simulink model "Spike_Generator_matt"  (R2019b)
settings: Solver=VariableStepAuto  StartTime=0.0  StopTime=testtime  RelTol=1e-3
InitFcn:
  | Spike_Generator_Test_Parameters
StopFcn:
  | Verify_Spike_Generator
values from neighbouring files (symbols this model uses):
  Fs = 48e3    (= 48000)    [Spike_Generator_Test_Parameters.m]    (also in modelparameters.m)
  nSites = 4    [Spike_Generator_Test_Parameters.m]
  tabs = 0.6e-3    (= 0.0006)    [Spike_Generator_Test_Parameters.m]
  trel = 0.6e-3    (= 0.0006)    [Spike_Generator_Test_Parameters.m]
libraries: dspsrcs4 x4
(part 2 of 3)

== stateflow chart Spike_Generator_matt/Spike Generator Singles/Stateflow Logic Chart ==
  settings: updateMethod=DISCRETE  sampleTime=tdres  executeAtInitialization=1
  note: 1st Synaptic Site State
      |
      | - Updates according to whether the synaptic site is sensing input or is going through the redocking period.
  note: 2nd Synaptic Site State
      |
      | - Updates according to whether the synaptic site is sensing input or is going through the redocking period.
  note: 3rd Synaptic Site State
      |
      | - Updates according to whether the synaptic site is sensing input or is going through the redocking period.
  note: 4th Synaptic Site State
      |
      | - Updates according to whether the synaptic site is sensing input or is going through the redocking period.
  note: Redocking Decay State
      |
      | - Updates according to whether the redocking period should be decayed or a redocking event has occured during the time step
  note: Synaptic State
      |
      | - Updates according to whether the synapse is ready to fire or is going through the refractory period.
  state SynapticSite1 [parallel]
    settings: executionOrder=2
    note: Synaptic Site Sensing Input
    note: Synaptic Site In Redocking Period
    note: Default Transition
    state SenseInput
      entry:
      SredockStatus1 = single(0);
      SXsum1 = SXsum1 + synout/(single(4));
      SreleaseStatus1 = checkRelease(SXsum1, SunitRateInterval1);
      during:
      SXsum1 = SXsum1 + synout/(single(4));
      SreleaseStatus1 = checkRelease(SXsum1, SunitRateInterval1);
      exit:
      SoneSiteRedock1 = getNewRedock(Scurrent_redocking_period, randNums);
      SXsum1= single(0);
      SunitRateInterval1 = getNewUnitRateInterval(randNums);
    state RedockPeriod
      entry:
      Selapsed_time1 = single(0);
      SredockStatus1 = checkRedock(Selapsed_time1, SoneSiteRedock1);
      Selapsed_time1  = Selapsed_time1 + Stdres;
      SreleaseStatus1 = single(0);
      during:
      SredockStatus1 = checkRedock(Selapsed_time1, SoneSiteRedock1);
      Selapsed_time1 = Selapsed_time1 + Stdres;
      exit:
      Selapsed_time1 = single(0);
      Scurrent_redocking_period = Sprevious_redocking_period + St_rd_jump;
      Sprevious_redocking_period = Scurrent_redocking_period;
    (default) -> SynapticSite1.RedockPeriod
    SynapticSite1.SenseInput -> SynapticSite1.RedockPeriod : [SreleaseStatus1 == single(1)]
    SynapticSite1.RedockPeriod -> SynapticSite1.SenseInput : [SredockStatus1 == single(1)]
  state SynapticSite2 [parallel]
    settings: executionOrder=3
    note: Synaptic Site Sensing Input
    note: Synaptic Site In Redocking Period
    note: Default Transition
    state SenseInput
      entry:
      SredockStatus2 = single(0);
      SXsum2 = SXsum2 + synout/(single(4));
      SreleaseStatus2 = checkRelease(SXsum2, SunitRateInterval2);
      during:
      SXsum2 = SXsum2 + synout/(single(4));
      SreleaseStatus2 = checkRelease(SXsum2, SunitRateInterval2);
      exit:
      SoneSiteRedock2 = getNewRedock(Scurrent_redocking_period, randNums);
      SXsum2= single(0);
      SunitRateInterval2 = getNewUnitRateInterval(randNums);
    state RedockPeriod
      entry:
      Selapsed_time2 = single(0);
      SredockStatus2 = checkRedock(Selapsed_time2, SoneSiteRedock2);
      Selapsed_time2  = Selapsed_time2 + Stdres;
      SreleaseStatus2 = single(0);
      during:
      SredockStatus2 = checkRedock(Selapsed_time2, SoneSiteRedock2);
      Selapsed_time2 = Selapsed_time2 + Stdres;
      exit:
      Selapsed_time2 = single(0);
      Scurrent_redocking_period = Sprevious_redocking_period + St_rd_jump;
      Sprevious_redocking_period = Scurrent_redocking_period;
    (default) -> SynapticSite2.RedockPeriod
    SynapticSite2.SenseInput -> SynapticSite2.RedockPeriod : [SreleaseStatus2 == single(1)]
    SynapticSite2.RedockPeriod -> SynapticSite2.SenseInput : [SredockStatus2 == single(1)]
  state SynapticSite3 [parallel]
    settings: executionOrder=4
    note: Synaptic Site Sensing Input
    note: Synaptic Site In Redocking Period
    note: Default Transition
    state SenseInput
      entry:
      SredockStatus3 = single(0);
      SXsum3 = SXsum3 + synout/(single(4));
      SreleaseStatus3 = checkRelease(SXsum3, SunitRateInterval3);
      during:
      SXsum3 = SXsum3 + synout/(single(4));
      SreleaseStatus3 = checkRelease(SXsum3, SunitRateInterval3);
      exit:
      SoneSiteRedock3 = getNewRedock(Scurrent_redocking_period, randNums);
      SXsum3= single(0);
      SunitRateInterval3 = getNewUnitRateInterval(randNums);
    state RedockPeriod
      entry:
      Selapsed_time3 = single(0);
      SredockStatus3 = checkRedock(Selapsed_time3, SoneSiteRedock3);
      Selapsed_time3  = Selapsed_time3 + Stdres;
      SreleaseStatus3 = single(0);
      during:
      SredockStatus3 = checkRedock(Selapsed_time3, SoneSiteRedock3);
      Selapsed_time3 = Selapsed_time3 + Stdres;
      exit:
      Selapsed_time3 = single(0);
      Scurrent_redocking_period = Sprevious_redocking_period + St_rd_jump;
      Sprevious_redocking_period = Scurrent_redocking_period;
    (default) -> SynapticSite3.RedockPeriod
    SynapticSite3.SenseInput -> SynapticSite3.RedockPeriod : [SreleaseStatus3 == single(1)]
    SynapticSite3.RedockPeriod -> SynapticSite3.SenseInput : [SredockStatus3 == single(1)]
  state SynapticSite4 [parallel]
    settings: executionOrder=5
    note: Synaptic Site Sensing Input
    note: Synaptic Site In Redocking Period
    note: Default Transition
    state SenseInput
      entry:
      SredockStatus4 = single(0);
      SXsum4 = SXsum4 + synout/(single(4));
      SreleaseStatus4 = checkRelease(SXsum4, SunitRateInterval4);
      during:
      SXsum4 = SXsum4 + synout/(single(4));
      SreleaseStatus4 = checkRelease(SXsum4, SunitRateInterval4);
      exit:
      SoneSiteRedock4 = getNewRedock(Scurrent_redocking_period, randNums);
      SXsum4= single(0);
      SunitRateInterval4 = getNewUnitRateInterval(randNums);
    state RedockPeriod
      entry:
      Selapsed_time4 = single(0);
      SredockStatus4 = checkRedock(Selapsed_time4, SoneSiteRedock4);
      Selapsed_time4  = Selapsed_time4 + Stdres;
      SreleaseStatus4 = single(0);
      during:
      SredockStatus4 = checkRedock(Selapsed_time4, SoneSiteRedock4);
      Selapsed_time4 = Selapsed_time4 + Stdres;
      exit:
      Selapsed_time4 = single(0);
      Scurrent_redocking_period = Sprevious_redocking_period + St_rd_jump;
      Sprevious_redocking_period = Scurrent_redocking_period;
    (default) -> SynapticSite4.RedockPeriod
    SynapticSite4.SenseInput -> SynapticSite4.RedockPeriod : [SreleaseStatus4 == single(1)]
    SynapticSite4.RedockPeriod -> SynapticSite4.SenseInput : [SredockStatus4 == single(1)]
  state RedockingDecay [parallel]
    settings: executionOrder=6
    note: Decay Redocking Period
    note: Don't Decay Redocking Period
    note: Default Transition
    state DecayRedockingPeriod
      entry:
      Scurrent_redocking_period = decayRedock(Sprevious_redocking_period, Stdres, Stau, St_rd_rest);
      Sprevious_redocking_period = Scurrent_redocking_period;
      Strd_vector = Scurrent_redocking_period;
      during:
      Scurrent_redocking_period = decayRedock(Sprevious_redocking_period, Stdres, Stau, St_rd_rest);
      Sprevious_redocking_period = Scurrent_redocking_period;
      Strd_vector = Scurrent_redocking_period;
    state NoDecay
      entry:
      Strd_vector = Scurrent_redocking_period;
      during:
      Strd_vector = Scurrent_redocking_period;
    (default) -> DecayRedockingPeriod
    DecayRedockingPeriod -> NoDecay : [SredockStatus1 == single(1) || SredockStatus2 == single(1) || SredockStatus3 == single(1) || SredockStatus4 == single(1)]
    NoDecay -> DecayRedockingPeriod : [SredockStatus1 == single(0) && SredockStatus2 == single(0) && SredockStatus3 == single(0) && SredockStatus4 == single(0)]
  state Synapse [parallel]
    settings: executionOrder=1
    note: Synapse Ready to Fire
    note: Synapse in Refractory Period
    note: Default Transition
    state RefractoryPeriod
      entry:
      SrefractoryStatus = checkRefractory(Srefractory_time, STref);
      Srefractory_time = Srefractory_time + Stdres;
      during:
      Ssptime = single(0);
      SrefractoryStatus = checkRefractory(Srefractory_time, STref);
      Srefractory_time = Srefractory_time + Stdres;
      exit:
      Srefractory_time = single(0);
      Ssptime = single(0);
    state SynapseReady
      during:
      Ssptime = single(0);
      exit:
      Ssptime = single(1);
      SspCount = SspCount + single(1);
      STref = getTref(synout, randNums, Strel, Stabs);
    (default) -> SynapseReady
    SynapseReady -> RefractoryPeriod : [SreleaseStatus1 == single(1) || SreleaseStatus2 == single(1) || SreleaseStatus3 == single(1) || SreleaseStatus4 == single(1)]
    RefractoryPeriod -> SynapseReady : [SrefractoryStatus == single(0)]
  note: Release Status Graphical Function
      |
      | Input : Sensing Input Sum (Xsum) & Release Threshold (unitRateInterval)
      |
      | Output : Release Status Condition (releaseStatus)
      |
      | - Checks if a Release Event Occurs for the Synaptic Site (1) or not (0)
  state releaseStatuscond = checkRelease(Xsumval, unitRateIntervalval) [function]
    (default) -> (junction 138) : % Check to see if a release event occurs.
    (junction 138) -> (junction 139) [order 1] : [Xsumval >= unitRateIntervalval]
    (junction 138) -> (junction 140) [order 2] : {releaseStatuscond = single(0);}
    (junction 139) -> (junction 141) : {releaseStatuscond = single(1);}
    (junction 141) -> (junction 140)
    (junction 140) -> (junction 142)
  state redockStatuscond = checkRedock(elapsed_timeval, oneSiteRedockval) [function]
    (default) -> (junction 153) : % Check to see if a redocking event occurs.
    (junction 153) -> (junction 154) [order 1] : [elapsed_timeval >= oneSiteRedockval]
    (junction 153) -> (junction 155) [order 2] : {redockStatuscond = single(0);}
    (junction 154) -> (junction 156) : {redockStatuscond = single(1);}
    (junction 156) -> (junction 155)
    (junction 155) -> (junction 157)
  note: Redock Status Graphical Function
      |
      | Input : Elapsed Time during Redocking Event (elapsed_time) & Site Specific Redocking Period (oneSiteRedock)
      |
      | Output : Redock Status Condition (redockStatus)
      |
      | - Checks if a Redocking Event Occurs for the Synaptic Site (1) or not (0)
  state refractoryStatuscond = checkRefractory(refractory_timeval, Trefval) [function]
    (default) -> (junction 272) : % Check to see if the synapse is in the refractory period.
    (junction 272) -> (junction 273) [order 1] : [refractory_timeval >= Trefval]
    (junction 272) -> (junction 274) [order 2] : {refractoryStatuscond = single(1);}
    (junction 273) -> (junction 275) : {refractoryStatuscond = single(0);}
    (junction 275) -> (junction 274)
    (junction 274) -> (junction 276)
  note: Refractory Status Graphical Function
      |
      | Input : Elapsed Time during Refractory Period (refractory_time) & Refractory Period (Tref)
      |
      | Output : Refractory Status Condition (refractoryStatus)
      |
      | - Checks if the Synapse is in the Refractory Period (1) or not (0)
  note: Get New Unit Rate Interval MATLAB Function
      |
      | Input : Uniformly Distributed Random Number between 0 and 1 (randNums)
      |
      | Output : New Release Threshold Value (unitRateInterval)
      |
      | - Calculates the New Release Threshold Value for the Synaptic Site after a Release Event
  note: Get New Site Specific Redocking Period MATLAB Function
      |
      | Input : Current Redocking Period (current_redocking_period) & Uniformly Distributed Random Number between 0 and 1 (randNums)
      |
      | Output : New Redocking Period for Specific Synaptic Site (oneSiteRedock)
      |
      | - Calculates the New Redocking Period for Specific Synaptic Site
  note: Decay Redocking Period MATLAB Function
      |
      | Input : Previous Redocking Period (previous_redocking_period), Sample Time (tdres),
      | Decay Time Constant (tau), & Resting Redocking Time (t_rd_rest)
      |
      | Output : Current Redocking Period (current_redocking_period)
      |
      | - Decays the Redocking Period for the Next TIme Step
  note: Get New Refractory Period MATLAB Function
      |
      | Input : Synapse Output (synout), Uniformly Distributed Random Number between 0 and 1 (randNums),
      | Relative Refractory Time (trel), & Absolute Refractory Time (tabs)
      |
      | Output : New Refractory Period for the Synapse (Tref)
      |
      | - Calculates the New Refractory Period for the Synapse
  data: Xsumval function_input single; releaseStatuscond function_output single; unitRateIntervalval function_input single; elapsed_timeval function_input single; redockStatuscond function_output single; oneSiteRedockval function_input single; refractory_timeval function_input single; refractoryStatuscond function_output single; Trefval function_input single; randNumsval function_input single; unitRateIntervalval function_output single; current_redocking_periodval function_input single; randNumsval function_input single; oneSiteRedockval function_output single; previous_redocking_periodval function_input single; current_redocking_periodval function_output single; tdresval function_input single; tauval function_input single; t_rd_restval function_input single; synoutval function_input single; Trefval function_output single; randNumsval function_input single; trelval function_input single; tabsval function_input single; Stdres parameter single; synout input single; SrefractoryStatus local single; randNums input single; Ssptime output single; SspCount output single; Scurrent_redocking_period output single; Strd_vector output single; St_rd_jump parameter single; SreleaseStatus1 local single; SredockStatus1 local single; SreleaseStatus4 local single; SredockStatus4 local single; SreleaseStatus2 local single; SredockStatus2 local single; SreleaseStatus3 local single; SredockStatus3 local single; St_rd_rest parameter single; Stau parameter single; Strel parameter single; Stabs parameter single; SunitRateInterval4 local single; SunitRateInterval3 local single; SunitRateInterval2 local single; SunitRateInterval1 local single; SoneSiteRedock4 local single; SoneSiteRedock3 local single; SoneSiteRedock2 local single; SoneSiteRedock1 local single; Selapsed_time4 local single; Selapsed_time3 local single; Selapsed_time2 local single; Selapsed_time1 local single; SXsum4 local single; SXsum3 local single; SXsum2 local single; SXsum1 local single; STref local single; Sprevious_redocking_period local single; Srefractory_time local single
  function unitRateIntervalval = getNewUnitRateInterval(randNumsval):
    | function unitRateIntervalval = getNewUnitRateInterval(randNumsval)
    |     unitRateIntervalval = single(-log(randNumsval)/Stdres);
    | end
  function oneSiteRedockval = getNewRedock(current_redocking_periodval, randNumsval):
    | function oneSiteRedockval = getNewRedock(current_redocking_periodval, randNumsval)
    |     oneSiteRedockval = single(-current_redocking_periodval * log(randNumsval));
    | end
  function current_redocking_periodval = decayRedock(previous_redocking_periodval,tdresval,tauval,t_rd_restval):
    | function current_redocking_periodval = decayRedock(previous_redocking_periodval,tdresval,tauval,t_rd_restval)
    |     current_redocking_periodval = single(previous_redocking_periodval - (tdresval/tauval)*(previous_redocking_periodval - t_rd_restval));
    | end
  function Trefval = getTref(synoutval, randNumsval, trelval, tabsval):
    | function Trefval = getTref(synoutval, randNumsval, trelval, tabsval)
    |     trel_k = min(trelval*100/synoutval,trelval);
    |     Trefval = single(tabsval - trel_k*log(randNumsval)); 
    | end
